simulink model "dVRK_RDOBS"  (Simulink 8.5)
settings: Solver=ode4  StartTime=0.0  StopTime=length(Tm)/1000  FixedStep=0.001  RelTol=1e-3
libraries: neural x630
(part 14 of 14)

== system dVRK_RDOBS/Joint 6 NN Dyn Ident/Layer 2/Delays 1 ==
  "p{2}" : Inport  PortDimensions=100  SampleTime=0.001
      mask Display: e = 0.06;c1 = [120 230 180]/255;c2 = ([120 230 180]+0)/(256+128);c3 = ([120 230 180]+128)/(256+128);patch([0 1 1 0],[0 0 1 1],c1);patch([0 1 1 1-e 1-e 0+e],[0 0 1 1-e 0+e 0+e],c2);patch([0 0 1 1-e 0+e 0+e],[0 1 1 1-e 1-e 0+e],c3);plot([0 1 1 0 0],[0 0 1 1 0]);
  mux : Mux  Inputs=1
      mask Display: e = 0.06;c1 = [120 150 230]/255;c2 = ([120 150 230]+0)/383;c3 = ([120 150 230]+128)/383;patch([0 1 1 0],[0 0 1 1],c1);patch([0 1 1 1-e 1-e 0+e],[0 0 1 1-e 0+e 0+e],c2);patch([0 0 1 1-e 0+e 0+e],[0 1 1 1-e 1-e 0+e],c3);plot([0 1 1 0 0],[0 0 1 1 0]);disp('Mux')
  "pd{2,1}" : Outport
      mask Display: e = 0.06;c1 = [120 230 180]/255;c2 = ([120 230 180]+0)/(256+128);c3 = ([120 230 180]+128)/(256+128);patch([0 1 1 0],[0 0 1 1],c1);patch([0 1 1 1-e 1-e 0+e],[0 0 1 1-e 0+e 0+e],c2);patch([0 0 1 1-e 0+e 0+e],[0 1 1 1-e 1-e 0+e],c3);plot([0 1 1 0 0],[0 0 1 1 0]);
  wires:
  "p{2}"/1 -> mux/1
  mux/1 -> "pd{2,1}"/1

== system dVRK_RDOBS/Joint 6 NN Dyn Ident/Layer 2/LW{2,1} ==
  "ad{2,1}" : Inport  PortDimensions=100  SampleTime=0.001
      mask Display: e = 0.06;c1 = [120 230 180]/255;c2 = ([120 230 180]+0)/(256+128);c3 = ([120 230 180]+128)/(256+128);patch([0 1 1 0],[0 0 1 1],c1);patch([0 1 1 1-e 1-e 0+e],[0 0 1 1-e 0+e 0+e],c2);patch([0 0 1 1-e 0+e 0+e],[0 1 1 1-e 1-e 0+e],c3);plot([0 1 1 0 0],[0 0 1 1 0]);
  "IW{2,1}(1,:)'" : Constant  Value=[-25.117904020399543;-2.9461298102710733;-0.37854026639176286;-0.24470136922249699;-0.45347189411314304;4.6515077008213819;-0.62340929388046684;-0.15923634300302875;-0.49603697179440048;-0.11527069068575008;0.3338445813829175;2.2591220040543463;-0.095144603884716725;2.358782342326164;-0.25627710026221134;-1.1486916466764856;0.18248968611056526;0.23461884166597574;0.46748487719341114;4.98971376349742;1.4180671849170008;5.3201668253840886;-0.14296081402472136;-0.18561403600665774;-1.6448061365653197;-10.016207250255926;-0.95841887068078491;-0.16122974532499279;0.5794415893120396;0.7552914591708576;2.0544904291203081;-0.29912739087887147;0.24449728730651971;12.292811376311974;0.21623795765123066;2.7335339069644595;0.25285897191017326;0.17078228982933025;0.47424527755556412;-0.24288329853253948;-0.31587244044582929;-3.1993144503220914;-1.1250447285229923;-0.55095021883430872;-0.1081048816039766;0.14608812122667589;0.15132093318519008;3.3175354978134983;1.7297494694514732;0.24904348718430064;-4.2565235620205382;-1.3862115148156837;0.15398629119947427;0.29095244449868746;0.20702840014947863;0.11351927081682006;-0.58391966948099461;0.11605532248457733;-0.42169905886316839;-0.21769982815102409;-5.411449245256855;0.4464330223891021;0.79831100878239081;-10.22014671927802;-0.18865526980149974;-1.0511692086937252;2.4611253437741749;0.9124818927682381;-5.4086052796658892;-0.41427865394871749;-6.6704195679358236;0.8110536446467298;-3.4011516602060818;0.14268371773143199;1.5564659921100095;2.6737616290335646;0.09569573071096335;0.65220456987785613;-2.2150937439133349;0.39747693092432002;-0.6982741799127421;-2.1606977400971457;0.26486939682074218;2.9186613831693267;0.14666745606708093;-3.5598903359810388;-0.19561100000702453;-0.79442179818465131;-0.46799940254342115;0.55259919900398236;0.71222840685675437;-0.34925946361388799;0.85517646074998643;0.95399631999332835;0.55845788702850518;-0.7467157928671071;6.1075020414851915;-6.4495486508851751;-4.1272389004241212;-0.11685923199950163]
      mask Display: e = 0.06;c1 = [120 150 230]/255;c2 = ([120 150 230]+0)/383;c3 = ([120 150 230]+128)/383;patch([0 1 1 0],[0 0 1 1],c1);patch([0 1 1 1-e 1-e 0+e],[0 0 1 1-e 0+e 0+e],c2);patch([0 0 1 1-e 0+e 0+e],[0 1 1 1-e 1-e 0+e],c3);plot([0 1 1 0 0],[0 0 1 1 0]);disp('weights');
  Mux : Mux  Inputs=1
      mask Display: e = 0.06;c1 = [120 150 230]/255;c2 = ([120 150 230]+0)/383;c3 = ([120 150 230]+128)/383;patch([0 1 1 0],[0 0 1 1],c1);patch([0 1 1 1-e 1-e 0+e],[0 0 1 1-e 0+e 0+e],c2);patch([0 0 1 1-e 0+e 0+e],[0 1 1 1-e 1-e 0+e],c3);plot([0 1 1 0 0],[0 0 1 1 0]);disp('Mux');
  dotprod1 : neural/Weight Functions/dotprod
  "lz{2,1}" : Outport
      mask Display: e = 0.06;c1 = [120 230 180]/255;c2 = ([120 230 180]+0)/(256+128);c3 = ([120 230 180]+128)/(256+128);patch([0 1 1 0],[0 0 1 1],c1);patch([0 1 1 1-e 1-e 0+e],[0 0 1 1-e 0+e 0+e],c2);patch([0 0 1 1-e 0+e 0+e],[0 1 1 1-e 1-e 0+e],c3);plot([0 1 1 0 0],[0 0 1 1 0]);
  wires:
  "IW{2,1}(1,:)'"/1 -> dotprod1/1
  "ad{2,1}"/1 -> dotprod1/2
  dotprod1/1 -> Mux/1
  Mux/1 -> "lz{2,1}"/1

== matlab function MATLAB Function2 ==
  data: J1 input double; Fext output double; T input double
function Fext = fcn(J1,T)
%#codegen
J=zeros(6,6);

J(1,1:6)=J1(1:6);
J(2,1:6)=J1(7:12);
J(3,1:6)=J1(13:18);
J(4,1:6)=J1(19:24);
J(5,1:6)=J1(25:30);
J(6,1:6)=J1(31:36);

Fext=inv(J')*T;
